simulink model "sh_testrig_accumulator_gas"  (R2019b)
settings: Solver=VariableStepAuto  StartTime=0.0  StopTime=12  MaxStep=0.24  RelTol=1e-3  EnableMultiTasking=on
undefined symbols (not defined in the file or in its folder): sigbuilder_block
libraries: fl_lib x5, nesl_utility x5, sh_lib x4
CloseFcn:
  | try,close(h1_sh_testrig_accumulator_gas),end
  | clear h1_sh_testrig_accumulator_gas
  | 
  | clear simlog_sh_testrig_accumulator_gas
Description:
  | Gas-Charged Accumulator Test Rig
settings Model: ExtModeAutoUpdateStatusClock=off  Creator=MathWorks  LastModifiedBy=remil
settings DataIOCC: LimitDataPoints=on  MaxDataPoints=10000  SaveFormat=Array  SignalLoggingSaveFormat=ModelDataLogs  ReturnWorkspaceOutputs=off  SignalLoggingName=logsout_sh_testrig_accumulator_gas
settings OptimizationCC: ExpressionDepthLimit=2147483647  InitFltsAndDblsToZero=on  LifeSpan=inf
settings DebuggingCC: SaveWithParameterizedLinksMsg=none  UnderspecifiedInitializationDetection=Classic  MergeDetectMultiDrivingBlocksExec=none  SignalResolutionControl=TryResolveAllWithWarning  SolverPrmCheckMsg=warning  MultiTaskDSMMsg=warning  MultiTaskCondExecSysMsg=none  FcnCallInpInsideContextMsg=warning  AllowSymbolicDim=off  StateNameClashWarn=warning  PregeneratedLibrarySubsystemCodeDiagnostic=none  SFUnexpectedBacktrackingDiag=warning  SFNoUnconditionalDefaultTransitionDiag=warning  SFExecutionAtInitializationDiag=none  ArithmeticOperatorsInVariantConditions=warning
settings HardwareCC: ProdBitPerPointer=32  ProdBitPerSizeT=32  ProdBitPerPtrDiffT=32  ProdLargestAtomicFloat=None  ProdIntDivRoundTo=Undefined  ProdEndianess=Unspecified  ProdWordSize=32  ProdHWDeviceType=32-bit Generic
settings ModelReferenceCC: PropagateSignalLabelsOutOfModel=off
settings SFSimCC: SimUseLocalCustomCode=off  CustomCodeUndefinedFunction=UseInterfaceOnly
settings RTWCC: RTWUseLocalCustomCode=off
settings CodeAppCC: StateflowObjectComments=on
settings GRTTargetCC: TargetFcnLib=ansi_tfl_tmw.mat  TargetLangStandard=C89/C90 (ANSI)  GeneratePreprocessorConditionals=Disable all  CombineOutputUpdateFcns=off  GRTInterface=on
settings ConfigComp: CovMetricSettings=dw  CovHtmlReporting=on  CovSaveCumulativeToWorkspaceVar=on  CovSaveSingleToWorkspaceVar=on  CovExternalEMLEnable=off  CovSFcnEnable=off
settings SimscapeCC: SimscapeLogType=all  SimscapeLogSimulationStatistics=on  SimscapeLogOpenViewer=on  SimscapeLogName=simlog_sh_testrig_accumulator_gas  SimscapeLogDataHistory=10000

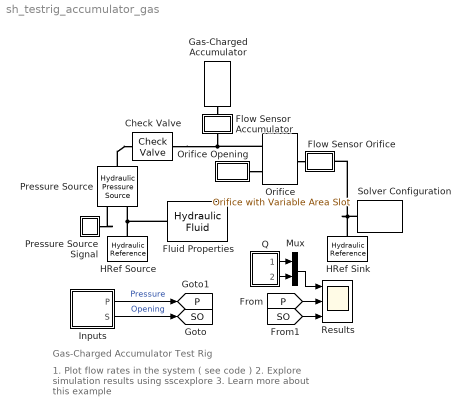
== system sh_testrig_accumulator_gas ==
  note: Gas-Charged Accumulator Test Rig
  note: 1. Plot flow rates in the system ( see code )
      | 2. Explore simulation results using sscexplore
      | 3. Learn more about this example
  Check Valve : sh_lib/Valves/Directional Valves/Check Valve  Tag=Factory Generic  area_max=0.0001 m^2  pres_crack=30000 Pa  pres_max=120000 Pa  C_d=0.7  A_leak=1e-12 m^2  lam_spec=1  B_lam=0.999  Re_cr=12  dynamic=0  tau=0.1 s  area_init=1e-12 m^2
      settings: SourceProductName=Simscape Fluids  SourceProductBaseCode=SH  InternalSimscapePortConfiguration="{\"Bottom\":[],\"Left\":[{\"id\":\"A\",\"label\":\"A\",\"type\":\"foundation.hydraulic.hydraulic\"}],\"Right\":[{\"id\":\"B\",\"label\":\"B\",\"type\":\"foundation.hydraulic.hydraulic\"}],\"Top\":[]}"
  Flow Sensor Accumulator : Subsystem
      mask Display: disp('QA')
  "Flow Sensor Orifice " : Subsystem
      mask Display: disp('QO');
  Fluid Properties : sh_lib/Hydraulic Utilities/Hydraulic Fluid  DataSource=1  SelFluid=1  SysTemp=60  TrapAir=0.005  ViscDerFactor=1  range_error=2
      settings: SourceProductName=Simscape Fluids
  Gas-Charged Accumulator : sh_lib/Accumulators/Gas-Charged Accumulator  capacity=8 l  dead_volume=0.08 l  pr_preload=5e5 Pa  k_sh=1.4  stiff_coeff=1e12 Pa/m^3  penetr_coeff=1e10 s*Pa/m^6  flow_rate_specify=off  flow_rate_priority=None  flow_rate=0.005 m^3/s  flow_rate_nominal_specify=off  flow_rate_nominal_unit=m^3/s  flow_rate_nominal_value=1  liquid_volume_specify=on  liquid_volume_priority=High  liquid_volume=1 l  liquid_volume_nominal_specify=off  liquid_volume_nominal_unit=m^3  liquid_volume_nominal_value=1  liquid_pressure_specify=off  liquid_pressure_priority=None  liquid_pressure=1.01325e+5 Pa  liquid_pressure_nominal_specify=off  liquid_pressure_nominal_unit=Pa  liquid_pressure_nominal_value=1
      settings: SourceProductName=Simscape Fluids  SourceProductBaseCode=SH  InternalSimscapePortConfiguration="{\"Bottom\":[],\"Left\":[],\"Right\":[{\"id\":\"A\",\"label\":\"A\",\"type\":\"foundation.hydraulic.hydraulic\"}],\"Top\":[]}"
  HRef Sink : fl_lib/Hydraulic/Hydraulic Elements/Hydraulic Reference  Tag=Factory Generic
      settings: SourceProductName=Simscape
  HRef Source : fl_lib/Hydraulic/Hydraulic Elements/Hydraulic Reference  Tag=Factory Generic
      settings: SourceProductName=Simscape
  "Inputs " : Subsystem  Tag=STV Subsys  LoadFcn=sigbuilder_block('load');  StartFcn=sigbuilder_block('start');  StopFcn=sigbuilder_block('stop');  ClipboardFcn=sigbuilder_block('clipboard');  mask(Sigbuilder block){tuvar=[0:10]}
      mask help: Sigbuilder GUI
      mask init:
      | if ~strcmp(get_param(bdroot(gcbh),'SimulationStatus'),'stopped') tuvar = sigbuilder_block('maskInit'); end
      settings: CopyFcn=sigbuilder_block('copy');  DeleteFcn=sigbuilder_block('delete');  ModelCloseFcn=sigbuilder_block('modelClose');  PreSaveFcn=sigbuilder_block('preSave');  PauseFcn=sigbuilder_block('pause')  ContinueFcn=sigbuilder_block('continue')  NameChangeFcn=sigbuilder_block('namechange');  OpenFcn=sigbuilder_block('open',[860.25 231 519.75 363 ]);  CloseFcn=sigbuilder_block('close');
      mask Display: plot(0, 0, 100, 100,[2, 2, 32, 32, 2], [68, 8, 8, 68, 68],[32, 2], [38, 38], [32, 19, 2],[53, 60, 44], [32, 17, 17, 2],[16, 16, 31, 31]);txt = getActiveGroup(gcbh);text(2, 100, txt,'verticalAlignment', 'top');
  Mux : Mux  Inputs=2
  Orifice : sh_lib/Orifices/Orifice with Variable Area Slot  Tag=Factory Generic  w=0.02 m  C_d=0.7  x_0=0 m  or=1  A_leak=1e-12 m^2  lam_spec=1  B_lam=0.999  Re_cr=12
      settings: SourceProductName=Simscape Fluids  SourceProductBaseCode=SH  InternalSimscapePortConfiguration="{\"Bottom\":[],\"Left\":[{\"id\":\"S\",\"label\":\"S\",\"type\":\"input\"},{\"id\":\"A\",\"label\":\"A\",\"type\":\"foundation.hydraulic.hydraulic\"}],\"Right\":[{\"id\":\"B\",\"label\":\"B\",\"type\":\"foundation.hydraulic.hydraulic\"}],\"Top\":[]}"
  Orifice Opening : Subsystem
      mask Display: disp('SO');
  Pressure Source : fl_lib/Hydraulic/Hydraulic Sources/Hydraulic Pressure Source  Tag=Factory Generic
      settings: SourceProductName=Simscape  SourceProductBaseCode=SS  InternalSimscapePortConfiguration="{\"Bottom\":[],\"Left\":[{\"id\":\"P\",\"label\":\"P\",\"type\":\"foundation.hydraulic.hydraulic\"}],\"Right\":[{\"id\":\"S\",\"label\":\"S\",\"type\":\"input\"},{\"id\":\"T\",\"label\":\"T\",\"type\":\"foundation.hydraulic.hydraulic\"}],\"Top\":[]}"
  Pressure Source Signal : Subsystem
      mask Display: disp('P')
  Q : Subsystem
  Results : Scope  NumInputPorts=3
  Solver Configuration : nesl_utility/Solver Configuration  PhysicalDomain=network_engine_domain  SubClassName=solver  LeftPortType=input  RightPortType=generic  Tones=[]  Harmonics=[]  SimulateNoise=off  Profile=off  UseLocalSampling=off  EnableSwitchedLinearOptims=on  FrequencyDomain=off  UseCCode=off  RelTol=0.001  AbsTol=1e-06  MinStep=1e-09  ToWorkspace=off  RevertToSquareIcSolve=off  NumHomotopyIterations=100  PhasorMode=off  PhasorModeNumHarmonics=1  DoDC=off  ResidualTolerance=1e-9  UseLocalSolver=off  LocalSolverChoice=NE_BACKWARD_EULER_ADVANCER  LocalSolverSampleTime=.001  DoFixedCost=off  MaxNonlinIter=3  MaxModeIter=2  LinearAlgebra=auto  EquationFormulation=NE_TIME_EF  DelaysMemoryBudget=1024  AutomaticFiltering=on  FilteringTimeConstant=0.001  PartitionStorageMethod=AS_NEEDED  PartitionMemoryBudget=1024  PartitionMethod=FAST
  tag scope: P=global, SO=global
  wires:
  "Inputs "/2(S) -> [SO]  "Opening"
  "Inputs "/1(P) -> [P]  "Pressure"
  [P] -> Results/2
  [SO] -> Results/3
  Mux/1 -> Results/1
  Q/1(QO) -> Mux/1
  Q/2(QA) -> Mux/2
  connections:
  Pressure Source/LConn1 -- Check Valve/LConn1
  HRef Source/LConn1 -- Fluid Properties/RConn1 -- Pressure Source/RConn2
  Orifice/LConn2 -- Flow Sensor Accumulator/LConn1 -- Check Valve/RConn1
  Gas-Charged Accumulator/RConn1 -- Flow Sensor Accumulator/RConn1
  Orifice/RConn1 -- "Flow Sensor Orifice "/LConn1
  HRef Sink/LConn1 -- Solver Configuration/RConn1 -- "Flow Sensor Orifice "/RConn1
  Orifice Opening/RConn1 -- Orifice/LConn1
  Pressure Source Signal/RConn1 -- Pressure Source/RConn1

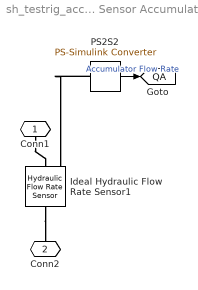
== system sh_testrig_accumulator_gas/Flow Sensor Accumulator ==
  Ideal Hydraulic Flow Rate Sensor1 : fl_lib/Hydraulic/Hydraulic Sensors/Hydraulic Flow Rate Sensor  Tag=Factory Generic
      settings: SourceProductName=Simscape
  PS2S2 : nesl_utility/PS-Simulink Converter  PhysicalDomain=network_engine_domain  SubClassName=ps_output  LeftPortType=input  RightPortType=output  PseudoPeriodic=off  Frequencies=[]  Unit=1  AffineConversion=off
  Conn1 : PMIOPort  Side=Right
  Conn2 : PMIOPort  Port=2  Side=Left
  tag scope: QA=global
  wires:
  PS2S2/1 -> [QA]  "Accumulator Flow Rate"
  connections:
  PS2S2/LConn1 -- Ideal Hydraulic Flow Rate Sensor1/RConn1
  Conn1/RConn1 -- Ideal Hydraulic Flow Rate Sensor1/RConn2
  Ideal Hydraulic Flow Rate Sensor1/LConn1 -- Conn2/RConn1

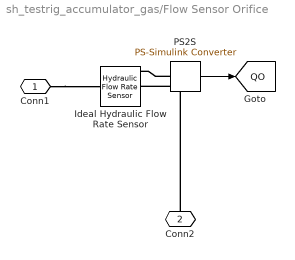
== system sh_testrig_accumulator_gas/Flow Sensor Orifice  ==
  Ideal Hydraulic Flow Rate Sensor : fl_lib/Hydraulic/Hydraulic Sensors/Hydraulic Flow Rate Sensor  Tag=Factory Generic
      settings: SourceProductName=Simscape
  PS2S : nesl_utility/PS-Simulink Converter  PhysicalDomain=network_engine_domain  SubClassName=ps_output  LeftPortType=input  RightPortType=output  PseudoPeriodic=off  Frequencies=[]  Unit=1  AffineConversion=off
  Conn1 : PMIOPort  Side=Left
  Conn2 : PMIOPort  Port=2  Side=Right
  tag scope: QO=global
  wires:
  PS2S/1 -> [QO]
  connections:
  PS2S/LConn1 -- Ideal Hydraulic Flow Rate Sensor/RConn1
  Conn2/RConn1 -- Ideal Hydraulic Flow Rate Sensor/RConn2
  Conn1/RConn1 -- Ideal Hydraulic Flow Rate Sensor/LConn1

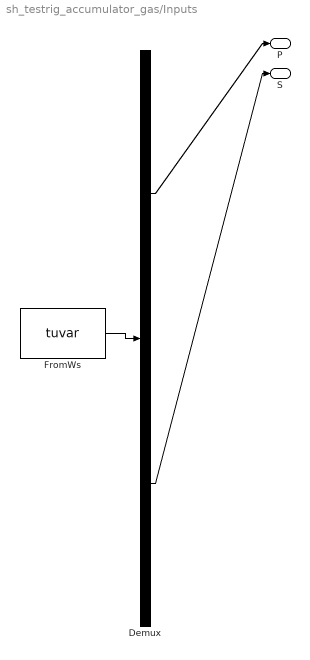
== system sh_testrig_accumulator_gas/Inputs  ==
  Demux : Demux  Tag=STV Demux  Outputs=2
  FromWs : FromWorkspace  Tag=STV FromWs  VariableName=tuvar  SampleTime=0
      SigBuilderData=|
      | common.afterFinalStr = 'Extrapolate'
      | common.sampleTime = 0
      | dataSet.timeRange = [0 12]
      | dataSet.name = 'Group 1'
      | sbobj.Groups.Name = 'Group 1'
      | sbobj.Groups.Signals(1).Name = 'P'
      | sbobj.Groups.Signals(1).XData = [0 0.2 2.8 3 6 6.2 8.8 9 12]
      | sbobj.Groups.Signals(1).YData = [500000 1000000 1000000 500000 500000 1000000 1000000 500000 500000]
      | sbobj.Groups.Signals(2).Name = 'S'
      | sbobj.Groups.Signals(2).XData = [0 3.5 3.7 5.3 5.5 9.5 9.7 11.3 11.5 12]
      | sbobj.Groups.Signals(2).YData = [0 0 0.005 0.00498 2e-05 0 0.00495 0.00495 0 0]
      | sbobj.Groups.TimeRange = [0 12]
  P : Outport  Tag=STV Outport  VectorParamsAs1DForOutWhenUnconnected=off
  S : Outport  Tag=STV Outport  Port=2  VectorParamsAs1DForOutWhenUnconnected=off
  wires:
  FromWs/1 -> Demux/1
  Demux/1 -> P/1
  Demux/2 -> S/1

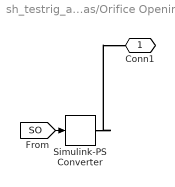
== system sh_testrig_accumulator_gas/Orifice Opening ==
  Simulink-PS Converter : nesl_utility/Simulink-PS Converter  PhysicalDomain=network_engine_domain  SubClassName=ps_input  LeftPortType=input  RightPortType=output  PseudoPeriodic=off  Frequencies=[]  NoiseDistribution=none  NoiseParameters=[]  Unit=1  AffineConversion=off  FilteringAndDerivatives=zero  SimscapeFilterOrder=1  InputFilterTimeConstant=.001  UdotUserProvided=0
  Conn1 : PMIOPort  Side=Right
  wires:
  [SO] -> Simulink-PS Converter/1
  connections:
  Simulink-PS Converter/RConn1 -- Conn1/RConn1

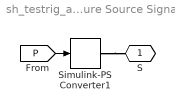
== system sh_testrig_accumulator_gas/Pressure Source Signal ==
  Simulink-PS Converter1 : nesl_utility/Simulink-PS Converter  PhysicalDomain=network_engine_domain  SubClassName=ps_input  LeftPortType=input  RightPortType=output  PseudoPeriodic=off  Frequencies=[]  NoiseDistribution=none  NoiseParameters=[]  Unit=1  AffineConversion=off  FilteringAndDerivatives=zero  SimscapeFilterOrder=1  InputFilterTimeConstant=.001  UdotUserProvided=0
  S : PMIOPort  Side=Right
  wires:
  [P] -> Simulink-PS Converter1/1
  connections:
  Simulink-PS Converter1/RConn1 -- S/RConn1

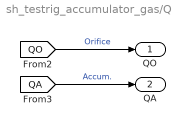
== system sh_testrig_accumulator_gas/Q ==
  QO : Outport  VectorParamsAs1DForOutWhenUnconnected=off
  QA : Outport  Port=2  VectorParamsAs1DForOutWhenUnconnected=off
  wires:
  [QA] -> QA/1  "Accum."
  [QO] -> QO/1  "Orifice"
